simulink model "conicaltank"  (R2021a)
settings: Solver=ode45  StartTime=0.0  StopTime=250  RelTol=1e-3  EnableMultiTasking=on
settings Model: Creator=Administrator  LastModifiedBy=Dell
settings SolverCC: AlgebraicLoopSolver=TrustRegion
settings DataIOCC: LimitDataPoints=on  SaveFormat=Array  ReturnWorkspaceOutputs=off
settings OptimizationCC: LifeSpan=inf
settings DebuggingCC: UnderspecifiedInitializationDetection=Classic  MergeDetectMultiDrivingBlocksExec=none  SolverPrmCheckMsg=warning  StateNameClashWarn=warning  SFUnexpectedBacktrackingDiag=warning  SFNoUnconditionalDefaultTransitionDiag=warning  SFExecutionAtInitializationDiag=none  SFMachineParentedDataDiag=warning  ArithmeticOperatorsInVariantConditions=warning
settings HardwareCC: ProdBitPerPointer=32  ProdBitPerSizeT=32  ProdBitPerPtrDiffT=32  ProdLargestAtomicFloat=None  ProdIntDivRoundTo=Undefined  ProdEndianess=Unspecified  ProdWordSize=32  ProdHWDeviceType=32-bit Generic
settings ModelReferenceCC: PropagateSignalLabelsOutOfModel=off
settings SFSimCC: SimUseLocalCustomCode=off  CustomCodeUndefinedFunction=UseInterfaceOnly
settings RTWCC: RTWUseLocalCustomCode=off
settings CodeAppCC: StateflowObjectComments=on
settings GRTTargetCC: TargetLangStandard=C89/C90 (ANSI)
settings ConfigComp: CovMetricSettings=dw  CovSaveCumulativeToWorkspaceVar=on  CovSaveSingleToWorkspaceVar=on  CovExternalEMLEnable=off

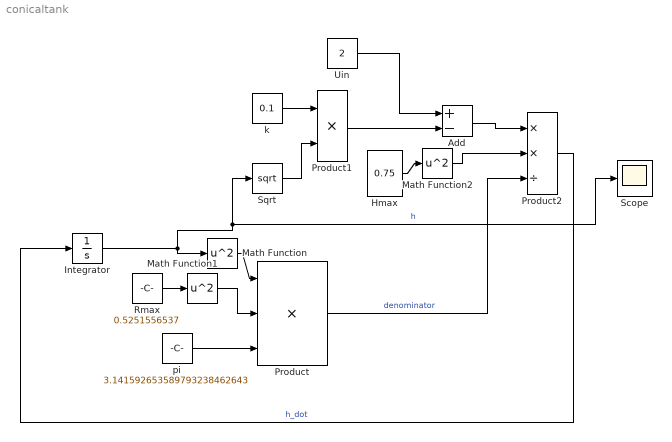
== system conicaltank ==
  Add : Sum  Inputs=+-
  Hmax : Constant  Value=0.75
  Integrator : Integrator  InitialCondition=0.25  LimitOutput=on  UpperSaturationLimit=0.75  LowerSaturationLimit=0
  Math Function : Math  Operator=square  SaturateOnIntegerOverflow=on
  Math Function1 : Math  Operator=square  SaturateOnIntegerOverflow=on
  Math Function2 : Math  Operator=square  SaturateOnIntegerOverflow=on
  Product : Product  Inputs=3
  Product1 : Product
  Product2 : Product  Inputs=**/
  Rmax : Constant  Value=0.5251556537
  Scope : Scope
  Sqrt : Sqrt  SaturateOnIntegerOverflow=on
  Uin : Constant  Value=2
  k : Constant  Value=0.1
  pi : Constant  Value=3.141592653589793238462643
  wires:
  Integrator/1 -> Math Function/1, Scope/1, Sqrt/1  "h"
  Product2/1 -> Integrator/1  "h_dot"
  Rmax/1 -> Math Function1/1
  k/1 -> Product1/1
  Sqrt/1 -> Product1/2
  Uin/1 -> Add/1
  Product1/1 -> Add/2
  Hmax/1 -> Math Function2/1
  Add/1 -> Product2/1
  Math Function/1 -> Product/1
  Math Function1/1 -> Product/2
  pi/1 -> Product/3
  Product/1 -> Product2/3  "denominator"
  Math Function2/1 -> Product2/2
